simulink model "Stabpendel_SignalAndScopeManager"  (Simulink 7.1)
settings: Solver=ode45  StartTime=0.0  StopTime=4.0  RelTol=1e-3
settings Model: Creator=Meisel  LastModifiedBy=Meisel

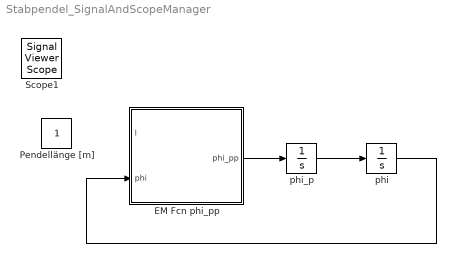
== system Stabpendel_SignalAndScopeManager ==
  EM Fcn phi_pp : Stateflow chart
  phi : Integrator  InitialCondition=30*pi/180
  phi_p : Integrator
  Pendellänge [m] : Constant  IOType=siggen  OutDataType=sfix(16)  OutScaling=2^0
  Scope1 : SignalViewerScope  IOType=viewer  RefreshTime=0.035000
  wires:
  phi_p/1 -> phi/1
  EM Fcn phi_pp/1(phi_pp) -> phi_p/1
  phi/1 -> EM Fcn phi_pp/2(phi)

== matlab function EM Fcn phi_pp ==
  data: l input double; phi_pp output double; phi input double
function phi_pp = fcn(l, phi)
% Embedded MATLAB 

phi_pp = 3/2*9.81 * sin(-phi) / l;
